simulink model "session"  (R2021a)
settings: Solver=VariableStepAuto  StartTime=0.0  StopTime=10.0  RelTol=1e-3
settings Model: Creator=Beshary  LastModifiedBy=Beshary

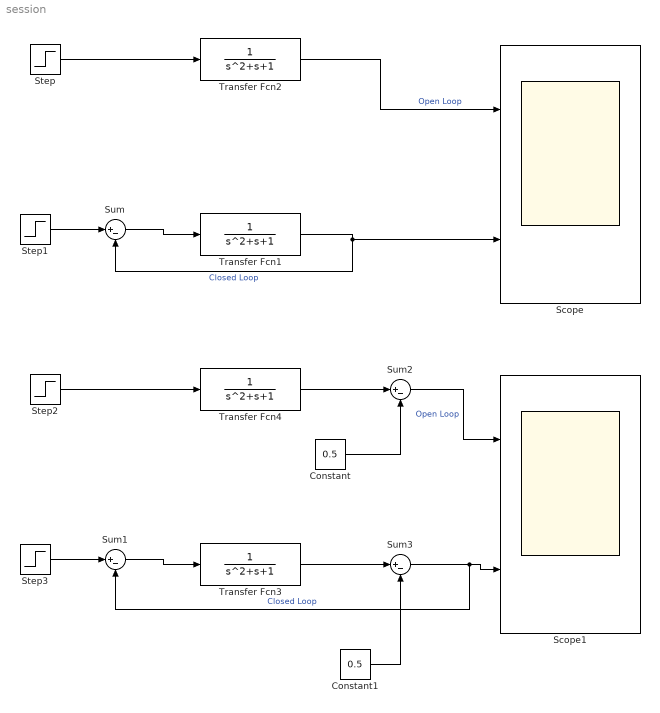
== system session ==
  Constant : Constant  Value=0.5
  Constant1 : Constant  Value=0.5
  Scope : Scope  NumInputPorts=2
  Scope1 : Scope  NumInputPorts=2
  Step{,1..3} (4 alike) : Step  SampleTime=0
  Sum{,1..3} (4 alike) : Sum  Inputs=|+-
  Transfer Fcn{1..4} (4 alike) : TransferFcn  Denominator=[1 1 1]
  wires:
  Step/1 -> Transfer Fcn2/1
  Transfer Fcn2/1 -> Scope/1  "Open Loop"
  Transfer Fcn1/1 -> Sum/2, Scope/2  "Closed Loop"
  Step1/1 -> Sum/1
  Sum/1 -> Transfer Fcn1/1
  Sum1/1 -> Transfer Fcn3/1
  Step3/1 -> Sum1/1
  Transfer Fcn4/1 -> Sum2/1
  Step2/1 -> Transfer Fcn4/1
  Sum2/1 -> Scope1/1  "Open Loop"
  Constant/1 -> Sum2/2
  Sum3/1 -> Scope1/2, Sum1/2  "Closed Loop"
  Constant1/1 -> Sum3/2
  Transfer Fcn3/1 -> Sum3/1
